simulink model "sistema_completo"  (R2019b)
settings: Solver=VariableStepAuto  StartTime=0.0  StopTime=1  RelTol=1e-3
libraries: powerlib x14, powerlib_meascontrol x1
settings Model: PacingRate=0.100000  Creator=Gabriel  LastModifiedBy=Gabriel
settings DataIOCC: ReturnWorkspaceOutputs=off

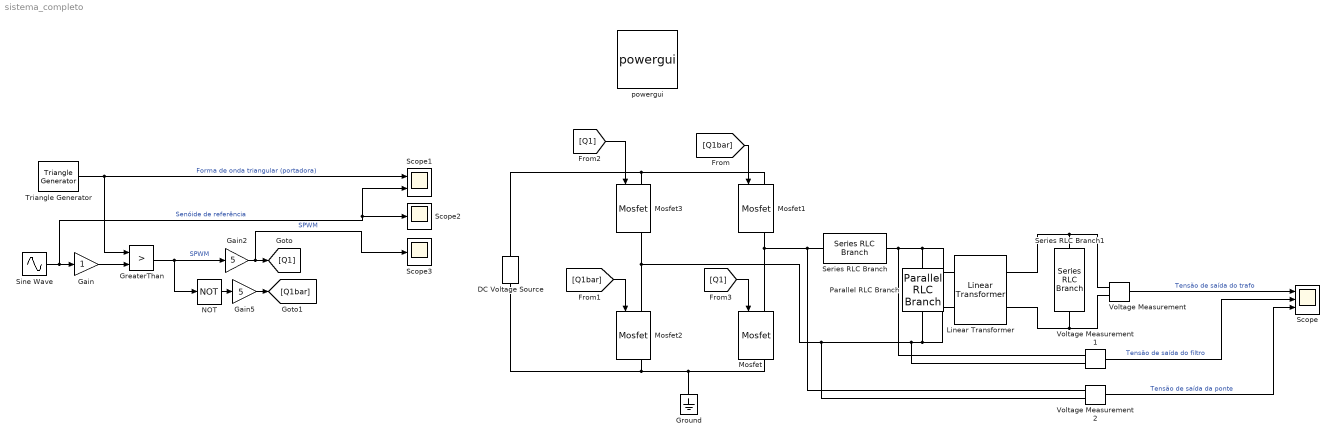
== system sistema_completo ==
  DC Voltage Source : powerlib/Electrical Sources/DC Voltage Source  Amplitude=12  Measurements=None
      settings: SourceProductName=Simscape Electrical
  Gain : Gain
  Gain2 : Gain  Gain=5
  Gain5 : Gain  Gain=5
  GreaterThan : RelationalOperator  Operator=>  OutDataTypeStr=boolean  RndMeth=Simplest
  Ground : powerlib/Elements/Ground  LConnTagsString=a
      settings: SourceProductName=Simscape Electrical
  Linear Transformer : powerlib/Elements/Linear Transformer  UNITS=SI  NominalPower=[ 50000 70 ]  winding1=[8.48 0.01 0]  winding2=[220 0.01 0]  ThreeWindings=off  winding3=[3.15e+05 0.7938 0.084225]  RmLm=[1e10 inf]  Measurements=None  DataType=on
      settings: SourceProductName=Simscape Electrical
  Mosfet{,1..3} (4 alike) : powerlib/Power Electronics/Mosfet  Ron=4.5e-3  Lon=0  Rd=0.01  Vfd=3.5  IC=0  Rs=inf  Cs=inf  Measurements=on
      settings: SourceProductName=Simscape Electrical
  NOT : Logic  Operator=NOT  IconShape=distinctive  AllPortsSameDT=off  OutDataTypeStr=boolean
  Parallel RLC Branch : powerlib/Elements/Parallel RLC Branch  LConnTagsString=a  RConnTagsString=__new0  BranchType=C  Resistance=500  Inductance=1e-3  SetiL0=off  InitialCurrent=0  Capacitance=470e-6  Setx0=off  InitialVoltage=0  Measurements=None
      settings: SourceProductName=Simscape Electrical
  Scope : Scope  NumInputPorts=3
  Scope1 : Scope  NumInputPorts=2
  Scope2 : Scope
  Scope3 : Scope
  Series RLC Branch : powerlib/Elements/Series RLC Branch  LConnTagsString=__new0  RConnTagsString=__new0  BranchType=L  Resistance=1  Inductance=2.4e-3  SetiL0=off  InitialCurrent=0  Capacitance=1e-6  Setx0=off  InitialVoltage=0  Measurements=None
      settings: SourceProductName=Simscape Electrical
  Series RLC Branch1 : powerlib/Elements/Series RLC Branch  LConnTagsString=__new0  RConnTagsString=__new0  BranchType=R  Resistance=1e4  Inductance=1e-3  SetiL0=off  InitialCurrent=0  Capacitance=1e-6  Setx0=off  InitialVoltage=0  Measurements=None
      settings: SourceProductName=Simscape Electrical
  Sine Wave : Sin  Frequency=2*pi*60  SampleTime=0
  Triangle Generator : powerlib_meascontrol/Pulse & Signal Generators/Triangle Generator  Freq=6e3  Phase=90  Ts=0
      settings: SourceProductName=Simscape Electrical
  Voltage Measurement : powerlib/Measurements/Voltage Measurement  PhasorSimulation=off  OutputType=Complex  PSBequivalent=0
      settings: SourceProductName=Simscape Electrical
  Voltage Measurement1 : powerlib/Measurements/Voltage Measurement  PhasorSimulation=off  OutputType=Complex  PSBequivalent=0
      settings: SourceProductName=Simscape Electrical
  Voltage Measurement2 : powerlib/Measurements/Voltage Measurement  PhasorSimulation=off  OutputType=Complex  PSBequivalent=0
      settings: SourceProductName=Simscape Electrical
  powergui : powerlib/powergui  Priority=1  SimulationMode=Continuous  SampleTime=50e-6  frequency=60  Iterations=50  frequencyindice=0  Pbase=100e6  ErrMax=1e-4  UnitsV=kV  UnitsW=MW  buscounter=0  FunctionMessages=off  echomessages=off  EnableUseOfTLC=off  CurrentSourceSwitches=off  DisableSnubberDevices=off  DisableRonSwitches=off  DisableVfSwitches=off  DisplayEquations=off  AutomaticDiscreteSolvers=off  SolverType=Tustin/Backward Euler (TBE)  Interpol=off  ExternalGateDelay=off  methode=off  Ts=100  x0status=blocks  SPID=on  SwTol=0  HookPort=off  NonlinearTolerance=1e-4  nMaxIteration=100  ContinueOnMaxIteration=off  RestoreLinks=warning  ResistiveCurrentMeasurement=off  Frange=[0:2:500]  Ylog=off  Xlog=on  ShowGrid=off  save=off  variable=ZData  structure=dados_inversor  ZoomFFT=off  StartTime=0.01  cycles=1  DisplayStyle=1  fundamental=60  FreqAxis=on  MaxFrequency=40000  frequencyindicesteady=1  RmsSteady=1  display=off
      settings: SourceProductName=Simscape Electrical
  wires:
  Sine Wave/1 -> Scope1/2, Scope2/1, Gain/1  "Senóide de referência"
  Gain/1 -> GreaterThan/2
  Triangle Generator/1 -> GreaterThan/1, Scope1/1  "Forma de onda triangular (portadora)"
  NOT/1 -> Gain5/1
  [Q1bar] -> Mosfet1/1
  [Q1] -> Mosfet3/1
  [Q1bar] -> Mosfet2/1
  [Q1] -> Mosfet/1
  Voltage Measurement1/1 -> Scope/2  "Tensão de saída do filtro"
  Voltage Measurement/1 -> Scope/1  "Tensão de saída do trafo"
  Voltage Measurement2/1 -> Scope/3  "Tensão de saída da ponte"
  GreaterThan/1 -> Gain2/1, NOT/1  "SPWM"
  Gain2/1 -> Scope3/1, [Q1]  "SPWM"
  Gain5/1 -> [Q1bar]
  connections:
  DC Voltage Source/LConn1 -- Mosfet/RConn1 -- Ground/LConn1 -- Mosfet2/RConn1
  Mosfet3/LConn1 -- DC Voltage Source/RConn1 -- Mosfet1/LConn1
  Mosfet1/RConn1 -- Mosfet/LConn1 -- Voltage Measurement2/LConn1 -- Series RLC Branch/LConn1
  Mosfet3/RConn1 -- Voltage Measurement2/LConn2 -- Voltage Measurement1/LConn2 -- Parallel RLC Branch/RConn1 -- Linear Transformer/LConn2 -- Mosfet2/LConn1
  Series RLC Branch/RConn1 -- Parallel RLC Branch/LConn1 -- Linear Transformer/LConn1 -- Voltage Measurement1/LConn1
  Series RLC Branch1/LConn1 -- Linear Transformer/RConn1 -- Voltage Measurement/LConn1
  Voltage Measurement/LConn2 -- Series RLC Branch1/RConn1 -- Linear Transformer/RConn2
